simulink model "Motors_PID_Simulink_Main"  (R2019b)
settings: Solver=VariableStepAuto  StartTime=0.0  StopTime=23  FixedStep=0.0001  RelTol=1e-3
undefined symbols (not defined in the file): desired_angle_vectors_drop1, desired_angle_vectors_drop2, desired_angle_vectors_drop3, desired_angle_vectors_m1, desired_angle_vectors_m2, desired_angle_vectors_m3, desired_angle_vectors_origin, EKb, EKm, EL, ER, GR, res, SKb, SKm, SL, SR, WKb, WKm, WL
libraries: cstblocks x4
settings Model: Creator=harsh  LastModifiedBy=harsh

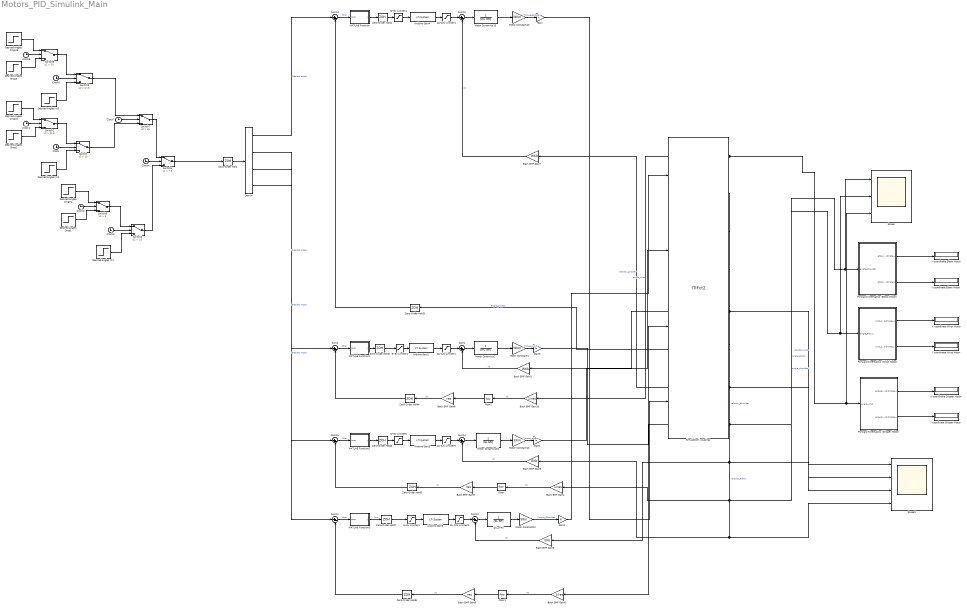
== system Motors_PID_Simulink_Main ==
  1/(Ls+R) : TransferFcn  Denominator=[SL SR]
  12/-12V Limiter{1,3..5} (4 alike) : Saturate  UpperLimit=12  LowerLimit=-12
  5/-5V Limiter{1,3..5} (4 alike) : Saturate  UpperLimit=5  LowerLimit=-5
  Arduino Gain1 : cstblocks/LTI System  sys=WOPAMP  IC=[]
  Arduino Gain3 : cstblocks/LTI System  sys=SOPAMP  IC=[]
  Arduino Gain4 : cstblocks/LTI System  sys=GOPAMP  IC=[]
  Arduino Gain5 : cstblocks/LTI System  sys=EOPAMP  IC=[]
  Back EMF Gain1 : Gain  Gain=WKb
  Back EMF Gain10 : Gain  Gain=1/res
  Back EMF Gain2 : Gain  Gain=1/res
  Back EMF Gain3 : Gain  Gain=res
  Back EMF Gain4 : Gain  Gain=1/res
  Back EMF Gain5 : Gain  Gain=res
  Back EMF Gain6 : Gain  Gain=res
  Back EMF Gain7 : Gain  Gain=WKb
  Back EMF Gain8 : Gain  Gain=SKb
  Back EMF Gain9 : Gain  Gain=EKb
  Clock{,1..7} (8 alike) : Clock
      settings: Decimation=100000
  Demux : Demux
  Desired Angles Drop1 : Step  Time=0.1  After=desired_angle_vectors_drop1  SampleTime=0
  Desired Angles Drop2 : Step  Time=0.1  After=desired_angle_vectors_drop2  SampleTime=0
  Desired Angles Drop3 : Step  Time=0.1  After=desired_angle_vectors_drop3  SampleTime=0
  Desired Angles Origin1 : Step  Time=0.1  After=desired_angle_vectors_origin  SampleTime=0
  Desired Angles Origin2 : Step  Time=0.1  After=desired_angle_vectors_origin  SampleTime=0
  Desired Angles Origin3 : Step  Time=0.1  After=desired_angle_vectors_origin  SampleTime=0
  Desired Angles m1 : Step  Time=0.1  After=desired_angle_vectors_m1  SampleTime=0
  "Desired Angles m2 " : Step  Time=0.1  After=desired_angle_vectors_m2  SampleTime=0
  Desired Angles m3 : Step  Time=0.1  After=desired_angle_vectors_m3  SampleTime=0
  Floor : Rounding
  Floor1 : Rounding
  Floor2 : Rounding
  Forward Kinematics (Elbow Motor) : MATLAB Function  TreatAsAtomicUnit=on
  Forward Kinematics (Gripper Motor) : MATLAB Function  TreatAsAtomicUnit=on
  Forward Kinematics (Wrist Motor) : MATLAB Function  TreatAsAtomicUnit=on
  Gain : Gain
  Gain1 : Gain  Gain=6
  Gain2 : Gain  Gain=6
  Gain3 : Gain  Gain=6
  MATLAB Function : MATLAB Function  TreatAsAtomicUnit=on
  MATLAB Function1 : MATLAB Function  TreatAsAtomicUnit=on
  MATLAB Function2 : MATLAB Function  TreatAsAtomicUnit=on
  MATLAB Function3 : MATLAB Function  TreatAsAtomicUnit=on
  Motor Constant1 : Gain  Gain=WKm
  Motor Constant10 : Gain  Gain=WKm
  Motor Constant12 : Gain  Gain=SKm
  Motor Constant13 : Gain  Gain=EKm
  Motor Dynamics13 : TransferFcn  Denominator=[WL GR]
  Motor Dynamics19 : TransferFcn  Denominator=[EL ER]
  Motor Dynamics2 : TransferFcn  Denominator=[WL GR]
  Scope : Scope  NumInputPorts=3
  Scope1 : Scope  NumInputPorts=4
  SimulationX coupling : S-Function  FunctionName=ITIFct2  Parameters=ip, port, ts, nIn, nOut  SFunctionDeploymentMode=off  EnableBusSupport=off  mask{ip='localhost', port=1026, ts=0.005, nIn=4, nOut=8}
      mask prompts: ip "Address: ip"; port "Port Number: port [-]"; ts "Communication Step Size: ts [s]"; nIn "Input Vector Dimension (to SimulationX): nIn [-]"; nOut "Output Vector Dimension (from SimulationX): nOut [-]"
      mask help: Coupling Element
  Sum{1..2,10..15} (8 alike) : Sum  Inputs=|+-
  Switch : Switch  Criteria=u2 > Threshold  Threshold=10
  Switch1 : Switch  Criteria=u2 > Threshold  Threshold=12.5
  Switch2 : Switch  Criteria=u2 > Threshold  Threshold=2.5
  Switch3 : Switch  Criteria=u2 > Threshold  Threshold=5
  Switch4 : Switch  Criteria=u2 > Threshold  Threshold=7.5
  Switch5 : Switch  Criteria=u2 > Threshold  Threshold=17.5
  Switch6 : Switch  Criteria=u2 > Threshold  Threshold=20
  Switch7 : Switch  Criteria=u2 > Threshold  Threshold=15
  X-coordinate Elbow Motor : Display
  X-coordinate Gripper Motor : Display
  X-coordinate Wrist Motor : Display
  Y coordinate Elbow Motor : Display
  Y coordinate Gripper Motor : Display
  Y coordinate Wrist Motor : Display
  Zero-Order Hold{,1,3..8} (8 alike) : ZeroOrderHold  SampleTime=0.0001
  Zero-Order Hold2 : ZeroOrderHold  SampleTime=-1
  wires:
  5/-5V Limiter4/1 -> Arduino Gain4/1
  Arduino Gain4/1 -> 12/-12V Limiter4/1
  Back EMF Gain7/1 -> Sum12/2  "Vb"
  Sum12/1 -> Motor Dynamics13/1
  Demux/1 -> Sum13/1  "Desired angle"
  12/-12V Limiter4/1 -> Sum12/1
  Motor Dynamics13/1 -> Motor Constant10/1  "I"
  Motor Constant10/1 -> Gain/1  "Torque_gripper"
  Sum13/1 -> MATLAB Function/1(error)  "Error"
  Sum2/1 -> MATLAB Function1/1(error)  "Error"
  12/-12V Limiter1/1 -> Sum1/1
  Motor Dynamics2/1 -> Motor Constant1/1  "I"
  Sum1/1 -> Motor Dynamics2/1
  5/-5V Limiter1/1 -> Arduino Gain1/1
  Back EMF Gain1/1 -> Sum1/2  "Vb"
  Arduino Gain1/1 -> 12/-12V Limiter1/1
  Demux/2 -> Sum2/1  "Desired angle"
  MATLAB Function2/1(y) -> Zero-Order Hold6/1
  Sum15/1 -> MATLAB Function2/1(error)  "Error"
  Motor Dynamics19/1 -> Motor Constant13/1  "I"
  Motor Constant13/1 -> Gain1/1  "Torque_elbow"
  12/-12V Limiter5/1 -> Sum14/1
  Sum14/1 -> Motor Dynamics19/1
  5/-5V Limiter5/1 -> Arduino Gain5/1
  Back EMF Gain9/1 -> Sum14/2  "Vb"
  Arduino Gain5/1 -> 12/-12V Limiter5/1
  Demux/3 -> Sum15/1  "Desired Angle"
  Back EMF Gain8/1 -> Sum10/2  "Vb"
  Motor Constant12/1 -> Gain2/1  "Torque_Shoulder"
  5/-5V Limiter3/1 -> Arduino Gain3/1
  Arduino Gain3/1 -> 12/-12V Limiter3/1
  1/(Ls+R)/1 -> Motor Constant12/1  "I"
  12/-12V Limiter3/1 -> Sum10/1
  MATLAB Function3/1(y) -> Zero-Order Hold7/1  "Tau"
  Sum11/1 -> MATLAB Function3/1(error)  "Error"
  Sum10/1 -> 1/(Ls+R)/1
  Demux/4 -> Sum11/1  "Desired Angle"
  MATLAB Function1/1(y) -> Zero-Order Hold2/1
  MATLAB Function/1(y) -> Zero-Order Hold1/1
  Zero-Order Hold/1 -> Demux/1
  Zero-Order Hold1/1 -> 5/-5V Limiter4/1
  Zero-Order Hold2/1 -> 5/-5V Limiter1/1
  Zero-Order Hold3/1 -> Sum13/2
  Zero-Order Hold4/1 -> Sum2/2
  Zero-Order Hold5/1 -> Sum15/2
  Zero-Order Hold6/1 -> 5/-5V Limiter5/1
  Zero-Order Hold7/1 -> 5/-5V Limiter3/1
  Zero-Order Hold8/1 -> Sum11/2
  SimulationX coupling/2 -> Scope1/1, Back EMF Gain1/1  "velocity_wrist"
  SimulationX coupling/1 -> Scope/3, Forward Kinematics (Gripper Motor)/1(angle_wrist), Back EMF Gain10/1  "angle_wrist"
  SimulationX coupling/3 -> Zero-Order Hold3/1  "angle_gripper"
  SimulationX coupling/4 -> Scope1/2, Back EMF Gain7/1  "velocity_gripper"
  Motor Constant1/1 -> Gain3/1  "Torque_wrist"
  SimulationX coupling/5 -> Back EMF Gain4/1, Scope/1, Forward Kinematics (Elbow Motor)/1(angle_shoulder)  "angle_shoulder"
  SimulationX coupling/6 -> Scope1/3, Back EMF Gain8/1  "velocity_shoulder"
  SimulationX coupling/7 -> Back EMF Gain2/1, Scope/2, Forward Kinematics (Wrist Motor)/1(angle_elbow)  "angle_elbow"
  SimulationX coupling/8 -> Scope1/4, Back EMF Gain9/1  "velocity_elbow"
  Gain/1 -> SimulationX coupling/4
  Gain1/1 -> SimulationX coupling/2
  Gain2/1 -> SimulationX coupling/1
  Gain3/1 -> SimulationX coupling/3
  Floor/1 -> Back EMF Gain3/1
  Back EMF Gain2/1 -> Floor/1  "Vb"
  Back EMF Gain3/1 -> Zero-Order Hold5/1  "Vb"
  Back EMF Gain4/1 -> Floor1/1  "Vb"
  Floor1/1 -> Back EMF Gain5/1
  Back EMF Gain5/1 -> Zero-Order Hold8/1  "Vb"
  Back EMF Gain6/1 -> Zero-Order Hold4/1  "Vb"
  Floor2/1 -> Back EMF Gain6/1
  Back EMF Gain10/1 -> Floor2/1  "Vb"
  Desired Angles Origin2/1 -> Switch1/1
  Desired Angles Drop3/1 -> Switch6/3
  Clock4/1 -> Switch4/2
  Switch5/1 -> Switch7/1
  Clock1/1 -> Switch1/2
  Switch6/1 -> Switch5/1
  Switch2/1 -> Switch4/3
  Desired Angles Drop1/1 -> Switch3/3
  Desired Angles m1/1 -> Switch2/3
  Switch1/1 -> Switch/1
  Clock6/1 -> Switch6/2
  Switch/1 -> Switch7/3
  Switch3/1 -> Switch2/1
  Clock2/1 -> Switch2/2
  Desired Angles Origin1/1 -> Switch3/1
  "Desired Angles m2 "/1 -> Switch/3
  Clock5/1 -> Switch5/2
  Clock/1 -> Switch/2
  Desired Angles Origin3/1 -> Switch6/1
  Desired Angles Drop2/1 -> Switch1/3
  Switch7/1 -> Switch4/1
  Clock3/1 -> Switch3/2
  Clock7/1 -> Switch7/2
  Desired Angles m3/1 -> Switch5/3
  Forward Kinematics (Elbow Motor)/1(elbow_coordinate_x) -> X-coordinate Elbow Motor/1
  Forward Kinematics (Elbow Motor)/2(elbow_coordinate_y) -> Y coordinate Elbow Motor/1
  Forward Kinematics (Wrist Motor)/2(wrist_coordinate_y) -> Y coordinate Wrist Motor/1
  Forward Kinematics (Wrist Motor)/1(wrist_coordinate_x) -> X-coordinate Wrist Motor/1
  Forward Kinematics (Gripper Motor)/1(gripper_coordinate_x) -> X-coordinate Gripper Motor/1
  Forward Kinematics (Gripper Motor)/2(gripper_coordinate_y) -> Y coordinate Gripper Motor/1
  Switch4/1 -> Zero-Order Hold/1

== matlab function Motors_PID_Simulink_Main/MATLAB Function1 ==
  settings: updateMethod=DISCRETE
  data: error input; y output
function y = fcn(error)

persistent previous_error;                  %previous error = current error for next iteration, initially set to 0;
persistent Ki_output;                        %need as persistent variable for Ki_output = Ki_output + (...)
persistent ept;                             %constant vector of exponentials (p*e^(-p*n*Ts)) where n = 1.....#of samples we want to average
persistent unweighted_differential_outputs;  %vector used for dot product with ept, shifted at each cycle. 

if isempty(previous_error)
    previous_error = 0;
end

%Trial values for testing against Built in PID block
Kp = 0.016;
Ki = 0.0000119;
Kd = 3.11914;

Ts = 0.0001;    %Controller frequency from Arduino assumed to be 10kHz.

%--------P controller part------------------
Kp_output = Kp*error;    

%---------I controller part-----------------

%Initializing Ki_output
if isempty(Ki_output)
    Ki_output = 0;
end

Ki_output = Ki_output + Ki*[(error + previous_error)/2]*Ts; %cumulative areas of trapeziums

%----------D controller part----------------
controlfreq = 10000; %Hz
filter_pole = 5000;  %big pole because we don't care much about averaging but we do care a lot about delay. (signal is not noisy)
n = 4*controlfreq/filter_pole;  %We are averaging 80 samples in this example


%Now, we initialize the ept vector (will remain constant valued throughout the program)
if isempty(ept)
    ept = zeros(1,n);
    for i = 1:n
        ept(i) = filter_pole*1.132*exp(-filter_pole*i*Ts);
    end
    %We want Ts*sum(ept) = 1 but this is not the case normally, so we have to scale the ept such that we get a sum
    %of 1. To account for discretization error, we scale it by multiplying it by 1.132 in this example. 
end

if isempty(unweighted_differential_outputs)
    unweighted_differential_outputs = zeros(1,n);
end 

unweighted_differential_outputs(1) = (error - previous_error); 
filtered_derivative = dot(ept,unweighted_differential_outputs);

Kd_output = Kd*filtered_derivative;

n2 = n+1; %n2 = 9
for count = 1:(n-1) %1:7 in this example
    unweighted_differential_outputs(n2-count) = unweighted_differential_outputs(n2 - count - 1);    %shift values by one index, and in next loop calculate one more new slope at index 1 (starting index)
end 

y = Kp_output + Ki_output + Kd_output;

previous_error = error; %this will help us move on to get new values for Ki and Kd

end

== matlab function Motors_PID_Simulink_Main/MATLAB Function ==
  settings: updateMethod=DISCRETE
  data: error input; y output
function y = fcn(error)

persistent previous_error;                  %previous error = current error for next iteration, initially set to 0;
persistent Ki_output;                        %need as persistent variable for Ki_output = Ki_output + (...)
persistent ept;                             %constant vector of exponentials (p*e^(-p*n*Ts)) where n = 1.....#of samples we want to average
persistent unweighted_differential_outputs;  %vector used for dot product with ept, shifted at each cycle. 

if isempty(previous_error)
    previous_error = 0;
end

%Trial values for testing against Built in PID block
Kp = 7.3697;
Ki = 24.525;
Kd = 0.04744;

Ts = 0.0001;    %Controller frequency from Arduino assumed to be 10kHz.

%--------P controller part------------------
Kp_output = Kp*error;    

%---------I controller part-----------------

%Initializing Ki_output
if isempty(Ki_output)
    Ki_output = 0;
end

Ki_output = Ki_output + Ki*[(error + previous_error)/2]*Ts; %cumulative areas of trapeziums

%----------D controller part----------------
controlfreq = 10000; %Hz
filter_pole = 5000;  %big pole because we don't care much about averaging but we do care a lot about delay. (signal is not noisy)
n = 4*controlfreq/filter_pole;  %We are averaging 80 samples in this example


%Now, we initialize the ept vector (will remain constant valued throughout the program)
if isempty(ept)
    ept = zeros(1,n);
    for i = 1:n
        ept(i) = filter_pole*1.132*exp(-filter_pole*i*Ts);
    end
    %We want Ts*sum(ept) = 1 but this is not the case normally, so we have to scale the ept such that we get a sum
    %of 1. To account for discretization error, we scale it by multiplying it by 1.132 in this example. 
end

if isempty(unweighted_differential_outputs)
    unweighted_differential_outputs = zeros(1,n);
end 

unweighted_differential_outputs(1) = (error - previous_error); 
filtered_derivative = dot(ept,unweighted_differential_outputs);

Kd_output = Kd*filtered_derivative;

n2 = n+1; %n2 = 9
for count = 1:(n-1) %1:7 in this example
    unweighted_differential_outputs(n2-count) = unweighted_differential_outputs(n2 - count - 1);    %shift values by one index, and in next loop calculate one more new slope at index 1 (starting index)
end 

y = Kp_output + Ki_output + Kd_output;

previous_error = error; %this will help us move on to get new values for Ki and Kd

end

== matlab function Motors_PID_Simulink_Main/MATLAB Function2 ==
  settings: updateMethod=DISCRETE
  data: error input; y output
function y = fcn(error)

persistent previous_error;                  %previous error = current error for next iteration, initially set to 0;
persistent Ki_output;                        %need as persistent variable for Ki_output = Ki_output + (...)
persistent ept;                             %constant vector of exponentials (p*e^(-p*n*Ts)) where n = 1.....#of samples we want to average
persistent unweighted_differential_outputs;  %vector used for dot product with ept, shifted at each cycle. 

if isempty(previous_error)
    previous_error = 0;
end

%Trial values for testing against Built in PID block
Kp = 0.015 %0.015;
Ki = 0.00001%0.000001;
Kd = 100%100;

Ts = 0.0001;    %Controller frequency from Arduino assumed to be 10kHz.

%--------P controller part------------------
Kp_output = Kp*error;    

%---------I controller part-----------------

%Initializing Ki_output
if isempty(Ki_output)
    Ki_output = 0;
end

Ki_output = Ki_output + Ki*[(error + previous_error)/2]*Ts; %cumulative areas of trapeziums

%----------D controller part----------------
controlfreq = 10000; %Hz
filter_pole = 5000;  %big pole because we don't care much about averaging but we do care a lot about delay. (signal is not noisy)
n = 4*controlfreq/filter_pole;  %We are averaging 80 samples in this example


%Now, we initialize the ept vector (will remain constant valued throughout the program)
if isempty(ept)
    ept = zeros(1,n);
    for i = 1:n
        ept(i) = filter_pole*1.132*exp(-filter_pole*i*Ts);
    end
    %We want Ts*sum(ept) = 1 but this is not the case normally, so we have to scale the ept such that we get a sum
    %of 1. To account for discretization error, we scale it by multiplying it by 1.132 in this example. 
end

if isempty(unweighted_differential_outputs)
    unweighted_differential_outputs = zeros(1,n);
end 

unweighted_differential_outputs(1) = (error - previous_error); 
filtered_derivative = dot(ept,unweighted_differential_outputs);

Kd_output = Kd*filtered_derivative;

n2 = n+1; %n2 = 9
for count = 1:(n-1) %1:7 in this example
    unweighted_differential_outputs(n2-count) = unweighted_differential_outputs(n2 - count - 1);    %shift values by one index, and in next loop calculate one more new slope at index 1 (starting index)
end 

y = Kp_output + Ki_output + Kd_output;

previous_error = error; %this will help us move on to get new values for Ki and Kd

end

== matlab function Motors_PID_Simulink_Main/MATLAB Function3 ==
  settings: updateMethod=DISCRETE
  data: error input; y output
function y = fcn(error)

persistent previous_error;                  %previous error = current error for next iteration, initially set to 0;
persistent Ki_output;                        %need as persistent variable for Ki_output = Ki_output + (...)
persistent ept;                             %constant vector of exponentials (p*e^(-p*n*Ts)) where n = 1.....#of samples we want to average
persistent unweighted_differential_outputs;  %vector used for dot product with ept, shifted at each cycle. 

if isempty(previous_error)
    previous_error = 0;
end

%Trial values for testing against Built in PID block
Kp = 0.46;
Ki = 0.0045;%0.45;
Kd = 0.06744;%0.06744;

Ts = 0.0001;    %Controller frequency from Arduino assumed to be 10kHz.

%--------P controller part------------------
Kp_output = Kp*error;    

%---------I controller part-----------------

%Initializing Ki_output
if isempty(Ki_output)
    Ki_output = 0;
end

Ki_output = Ki_output + Ki*[(error + previous_error)/2]*Ts; %cumulative areas of trapeziums

%----------D controller part----------------
controlfreq = 10000; %Hz
filter_pole = 5000;  %big pole because we don't care much about averaging but we do care a lot about delay. (signal is not noisy)
n = 4*controlfreq/filter_pole;  %We are averaging 80 samples in this example


%Now, we initialize the ept vector (will remain constant valued throughout the program)
if isempty(ept)
    ept = zeros(1,n);
    for i = 1:n
        ept(i) = filter_pole*1.132*exp(-filter_pole*i*Ts);
    end
    %We want Ts*sum(ept) = 1 but this is not the case normally, so we have to scale the ept such that we get a sum
    %of 1. To account for discretization error, we scale it by multiplying it by 1.132 in this example. 
end

if isempty(unweighted_differential_outputs)
    unweighted_differential_outputs = zeros(1,n);
end 

unweighted_differential_outputs(1) = (error - previous_error); 
filtered_derivative = dot(ept,unweighted_differential_outputs);

Kd_output = Kd*filtered_derivative;

n2 = n+1; %n2 = 9
for count = 1:(n-1) %1:7 in this example
    unweighted_differential_outputs(n2-count) = unweighted_differential_outputs(n2 - count - 1);    %shift values by one index, and in next loop calculate one more new slope at index 1 (starting index)
end 

y = Kp_output + Ki_output + Kd_output;

previous_error = error; %this will help us move on to get new values for Ki and Kd

end

== matlab function Motors_PID_Simulink_Main/Forward Kinematics (Elbow Motor) ==
  data: angle_shoulder input; elbow_coordinate_x output; elbow_coordinate_y output
function [elbow_coordinate_x, elbow_coordinate_y] = fcn(angle_shoulder)
angle_shoulder_deg = rad2deg(angle_shoulder);

% If the input angle is negative, make it positive for analysis by adding 360
if angle_shoulder_deg < 0
    angle_shoulder_deg = 360 + angle_shoulder_deg;
end

%conditional statements for obtaining the coordinates of the elbow and wrist motors from the angle traversed
if angle_shoulder_deg < 90
    elbow_coordinate_x = 5*cosd(angle_shoulder_deg);
    elbow_coordinate_y = 5*sind(angle_shoulder_deg);
    
elseif 90 < angle_shoulder_deg && angle_shoulder_deg < 180 %2nd quadrant - x coordinates are negative
    elbow_coordinate_x = -5*cosd(180 - angle_shoulder_deg);
    elbow_coordinate_y = 5*sind(180 - angle_shoulder_deg);
        
elseif 180 < angle_shoulder_deg && angle_shoulder_deg < 270 %3rd quadrant - x coordinates are negative
    elbow_coordinate_x = -5*cosd(angle_shoulder_deg - 180);
    elbow_coordinate_y = 5*sind(angle_shoulder_deg - 180);
   
else                                                        %4th quadrant - x coordinates are negative
    elbow_coordinate_x = 5*cosd(360 - angle_shoulder_deg);
    elbow_coordinate_y = -5*sind(360 - angle_shoulder_deg);    
end

end

== matlab function Motors_PID_Simulink_Main/Forward Kinematics (Wrist Motor) ==
  data: angle_elbow input; wrist_coordinate_x output; wrist_coordinate_y output
function [wrist_coordinate_x, wrist_coordinate_y] = fcn(angle_elbow)
angle_elbow_deg = rad2deg(angle_elbow);

% If the input angle is negative, make it positive for analysis by adding 360
if angle_elbow_deg < 0
    angle_elbow_deg = 360 + angle_elbow_deg;
end

%conditional statements for obtaining the coordinates of the elbow and wrist motors from the angle traversed
if angle_elbow_deg < 90
    wrist_coordinate_x = 4*cosd(angle_elbow_deg);
    wrist_coordinate_y = 4*sind(angle_elbow_deg);
    
elseif 90 < angle_elbow_deg && angle_elbow_deg < 180 %2nd quadrant - x coordinates are negative
    wrist_coordinate_x = -4*cosd(180 - angle_elbow_deg);
    wrist_coordinate_y = 4*sind(180 - angle_elbow_deg);
        
elseif 180 < angle_elbow_deg && angle_elbow_deg < 270 %3rd quadrant - x coordinates are negative
    wrist_coordinate_x = -4*cosd(angle_elbow_deg - 180);
    wrist_coordinate_y = 4*sind(angle_elbow_deg - 180);
   
else                                                        %4th quadrant - x coordinates are negative
    wrist_coordinate_x = 4*cosd(360 - angle_elbow_deg);
    wrist_coordinate_y = -4*sind(360 - angle_elbow_deg);    
end

end

== matlab function Motors_PID_Simulink_Main/Forward Kinematics (Gripper Motor) ==
  data: angle_wrist input; gripper_coordinate_x output; gripper_coordinate_y output
function [gripper_coordinate_x, gripper_coordinate_y] = fcn(angle_wrist)
angle_wrist_deg = rad2deg(angle_wrist);

% If the input angle is negative, make it positive for analysis by adding 360
if angle_wrist_deg < 0
    angle_wrist_deg = 360 + angle_wrist_deg;
end

%conditional statements for obtaining the coordinates of the elbow and wrist motors from the angle traversed
if angle_wrist_deg < 90
    gripper_coordinate_x = 1*cosd(angle_wrist_deg);
    gripper_coordinate_y = 1*sind(angle_wrist_deg);
    
elseif 90 < angle_wrist_deg && angle_wrist_deg < 180 %2nd quadrant - x coordinates are negative
    gripper_coordinate_x = -1*cosd(180 - angle_wrist_deg);
    gripper_coordinate_y = 1*sind(180 - angle_wrist_deg);
        
elseif 180 < angle_wrist_deg && angle_wrist_deg < 270 %3rd quadrant - x coordinates are negative
    gripper_coordinate_x = -1*cosd(angle_wrist_deg - 180);
    gripper_coordinate_y = 1*sind(angle_wrist_deg - 180);
   
else                                                        %4th quadrant - x coordinates are negative
    gripper_coordinate_x = 1*cosd(360 - angle_wrist_deg);
    gripper_coordinate_y = -1*sind(360 - angle_wrist_deg);    
end

end
